simulink model "Kalman_offline"  (R2022b)
settings: Solver=VariableStepAuto  StartTime=0.0  StopTime=10.0  RelTol=1e-3
values from neighbouring files (symbols this model uses):
  A_d = (eye(size(A))+Ts*A)    [Kalman_offline.m]    (also in Main_sim.m; Startup_Script.m; Startup_labview.m; Test_ss.m)
  B_d = Ts*B    [Kalman_offline.m]    (also in Main_sim.m; Startup_Script.m; Startup_labview.m; Test_ss.m)
  bike_params = LoadBikeParameters(bike)    [Kalman_offline.m]    (also in Main_sim.m; Startup_Script.m; Startup_Script_v2.m; Startup_labview.m)
  C1 = [1 0 0 0 0 0 0 ... (first row only)    [Kalman_offline.m]    (also in Main_sim.m; Startup_Script.m; Startup_labview.m)
  C2 = [g+((-h_imu*g)/h) 0 (-h_imu*(h*v^2-(g*lr*c)))*sin(lambda)/((lr+lf)*h^2) + (v^2)*sin(lambda)/(lr+lf) 0 ... (first row only)    [Kalman_offline.m]    (also in Main_sim.m = [(-g+((-h_imu*g)/h)) 0 (-h_imu*(h*v^2-(g*lr*c)))*sin(lambda); Startup_Script.m = [(-g+((-h_imu*g)/h)) 0 (-h_imu*(h*v^2-(g*lr*c)))*sin(lambda); Startup_labview.m = [(g+((-h_imu*g)/h)) 0 (-h_imu*(h*v^2-(g*lr*c)))*sin(lambda)/)
  counter = (Ts_GPS / Ts) - 1    (= 9)    [Kalman_offline.m]    (also in Main_sim.m; Startup_Script.m; Startup_labview.m)
  D1 = [0 0 (-h_imu*lr*v)*sin(lambda)/((lr+lf)*h) 0 0 0 0]'    [Kalman_offline.m]    (also in Main_sim.m = [0 0 (-h_imu*lr*v)/((lr+lf)*h) 0 0 0 0]'; Startup_Script.m = [0 0 (-h_imu*lr*v)/((lr+lf)*h) 0 0 0 0]'; Startup_labview.m = [0 0 (-h_imu*lr*v)/((lr+lf)*h) 0 0 0 0]')
  D2 = [(-h_imu*lr*v)*sin(lambda)/((lr+lf)*h) 0 0 0 0]'    [Kalman_offline.m]    (also in Main_sim.m = [(-h_imu*lr*v)/((lr+lf)*h) 0 0 0 0]'; Startup_Script.m = [(-h_imu*lr*v)/((lr+lf)*h) 0 0 0 0]'; Startup_labview.m = [(-h_imu*lr*v)/((lr+lf)*h) 0 0 0 0]')
  initial_state_estimate = initial_state    [Main_sim.m]    (also in Startup_Script.m; Startup_Script_v2.m)
  Kalman_gain1 = Kalman_gain1'    [Kalman_offline.m]    (also in Main_sim.m; Startup_Script.m; Startup_labview.m)
  Kalman_gain2 = Kalman_gain2'    [Kalman_offline.m]    (also in Main_sim.m = Kalman_gain1(4:7,3:7); Startup_Script.m; Startup_labview.m = Kalman_gain1(4:7,3:7))
  lambda = bike_params.lambda_mod    [Kalman_offline.m]    (also in Main_sim.m; Startup_Script.m; Startup_Script_v2.m = bike_params.lambda; Startup_labview.m = bike_params.lambda)
  T = Rz*Ry*Rx    [Main_sim.m]    (also in Startup_Script.m)
  Ts = 0.01    [Kalman_offline.m]    (also in Main_sim.m; Startup_Script.m; Startup_Script_v2.m; Startup_labview.m)
  v = 3    [Main_sim.m]    (also in Startup_Script.m; Startup_Script_v2.m; Startup_labview.m = 2; Test_ss.m)
undefined symbols (not defined in the file or in its folder): initial_state
libraries: simulink x1
settings Model: Creator=gaizk  LastModifiedBy=gaizk

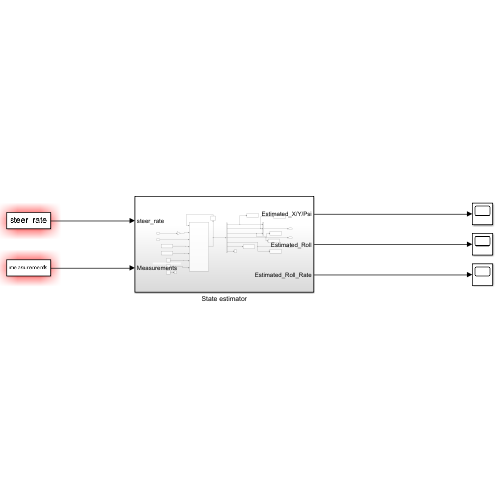
[thumbnail: Simulink's stored preview of the top-level diagram]
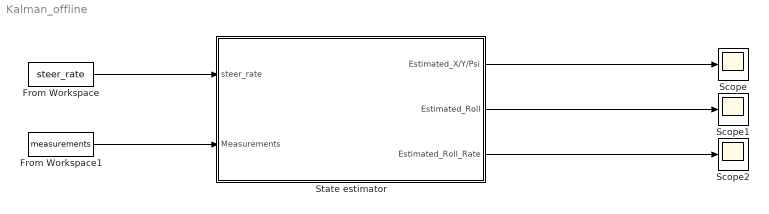
== system Kalman_offline ==
  From Workspace : FromWorkspace  VariableName=steer_rate
  From Workspace1 : FromWorkspace  VariableName=measurements
  Scope : Scope
  Scope1 : Scope
  Scope2 : Scope
  State estimator : Subsystem
  wires:
  From Workspace/1 -> State estimator/1(steer_rate)
  State estimator/1(Estimated_X/Y/Psi) -> Scope/1
  State estimator/2(Estimated_Roll) -> Scope1/1
  State estimator/3(Estimated_Roll_Rate) -> Scope2/1
  From Workspace1/1 -> State estimator/2(Measurements)

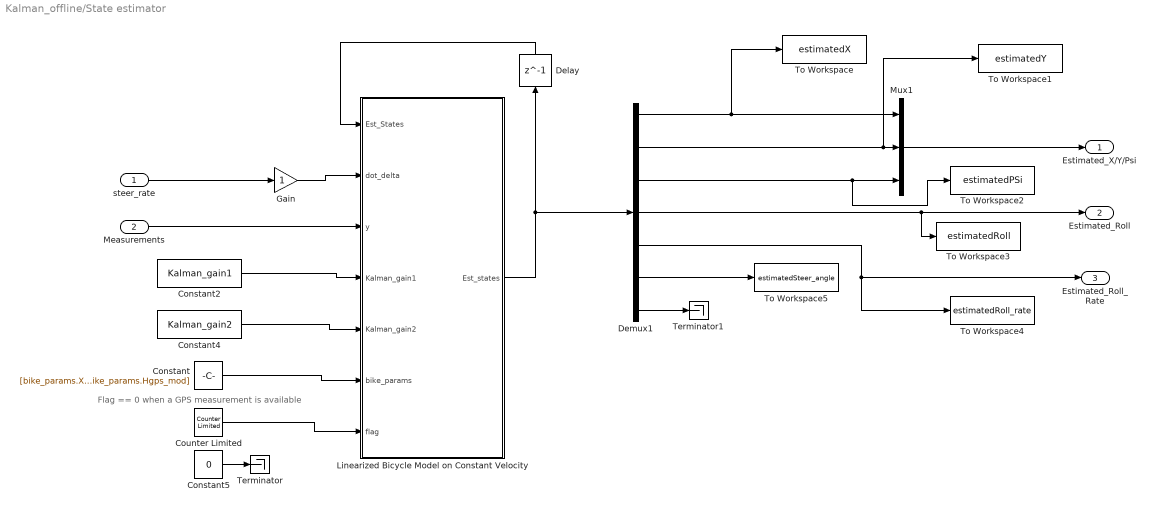
== system Kalman_offline/State estimator ==
  note: Flag == 0 when a GPS measurement is available
  steer_rate : Inport
  Measurements : Inport  Port=2
  Constant : Constant  Value=[bike_params.Xgps_mod bike_params.Ygps_mod bike_params.Hgps_mod]
  Constant2 : Constant  Value=Kalman_gain1  SampleTime=Ts
  Constant4 : Constant  Value=Kalman_gain2  SampleTime=Ts
  Constant5 : Constant  Value=0
  Counter Limited : simulink/Sources/Counter Limited  uplimit=counter  tsamp=Ts
  Delay : Delay  DelayLength=1  InitialCondition=[initial_state_estimate.x initial_state_estimate.y initial_state_estimate.heading initial_state.roll initial_state.roll_rate initial_state.steering v]  SampleTime=Ts
  Demux1 : Demux  Outputs=7
  Gain : Gain
  Linearized Bicycle Model on Constant Velocity : MATLAB Function  TreatAsAtomicUnit=on
  Mux1 : Mux  Inputs=3
  Terminator : Terminator
  Terminator1 : Terminator
  To Workspace : ToWorkspace  VariableName=estimatedX  SaveFormat=Timeseries  SampleTime=-1
  To Workspace1 : ToWorkspace  VariableName=estimatedY  SaveFormat=Timeseries  SampleTime=-1
  To Workspace2 : ToWorkspace  VariableName=estimatedPSi  SaveFormat=Timeseries  SampleTime=-1
  To Workspace3 : ToWorkspace  VariableName=estimatedRoll  SaveFormat=Timeseries  SampleTime=-1
  To Workspace4 : ToWorkspace  VariableName=estimatedRoll_rate  SaveFormat=Timeseries  SampleTime=-1
  To Workspace5 : ToWorkspace  VariableName=estimatedSteer_angle  SaveFormat=Timeseries  SampleTime=-1
  Estimated_X/Y/Psi : Outport  VectorParamsAs1DForOutWhenUnconnected=off
  Estimated_Roll : Outport  Port=2  VectorParamsAs1DForOutWhenUnconnected=off
  Estimated_Roll_Rate : Outport  Port=3  VectorParamsAs1DForOutWhenUnconnected=off
  wires:
  Linearized Bicycle Model on Constant Velocity/1(Est_states) -> Delay/1, Demux1/1
  Gain/1 -> Linearized Bicycle Model on Constant Velocity/2(dot_delta)
  Demux1/6 -> To Workspace5/1
  Demux1/5 -> Estimated_Roll_Rate/1, To Workspace4/1
  Delay/1 -> Linearized Bicycle Model on Constant Velocity/1(Est_States)
  steer_rate/1 -> Gain/1
  Demux1/2 -> To Workspace1/1, Mux1/2
  Demux1/1 -> To Workspace/1, Mux1/1
  Demux1/7 -> Terminator1/1
  Mux1/1 -> Estimated_X/Y/Psi/1
  Demux1/4 -> Estimated_Roll/1, To Workspace3/1
  Constant2/1 -> Linearized Bicycle Model on Constant Velocity/4(Kalman_gain1)
  Constant4/1 -> Linearized Bicycle Model on Constant Velocity/5(Kalman_gain2)
  Counter Limited/1 -> Linearized Bicycle Model on Constant Velocity/7(flag)
  Demux1/3 -> To Workspace2/1, Mux1/3
  Constant5/1 -> Terminator/1
  Constant/1 -> Linearized Bicycle Model on Constant Velocity/6(bike_params)
  Measurements/1 -> Linearized Bicycle Model on Constant Velocity/3(y)

== matlab function Kalman_offline/State estimator/Linearized Bicycle Model on Constant Velocity ==
  data: Est_States input; dot_delta input; y input; Kalman_gain1 input; Kalman_gain2 input; bike_params input; Est_states output; flag input; A_d parameter; B_d parameter; C1 parameter; C2 parameter; D1 parameter; D2 parameter; lambda parameter; T parameter
function Est_states  = fcn(Est_States, dot_delta, y, Kalman_gain1, Kalman_gain2, bike_params, flag, A_d, B_d, C1, C2, D1, D2, lambda, T)
% description 
% Inputs
%   Est_States := [X Y psi phi phi_dot delta v] are global at time t 
%   dot_delta_e := effective steering rate
%   y := measurement vector
%   Kalman_gain1 := Computed state_feedback gain including GPS meas
%   Kalman_gain2 := Computed state_feedback gain excluding GPS meas
%   bike_params := vector of bike parameters + gravity
%   Ts := Estimator sampling rate
%   v := constant velocity
%   flag := [0-1] increasing counter reseted at 1. When flag == 0 means
%           that GPS measurement is available
%
% Outputs
%   Est_states : = [X Y psi phi phi_dot delta v] global at time t+1


% Transform the states to local frame 
    Est_States_l = zeros(7,1);
    
    Est_States_l(1) = Est_States(1) * cos(Est_States(3)) + Est_States(2) * sin(Est_States(3));
    Est_States_l(2) = -Est_States(1) * sin(Est_States(3)) + Est_States(2) * cos(Est_States(3));
    Est_States_l(3) = 0;        % direction of bike is aligned with X local frame
    Est_States_l(4) = Est_States(4);
    Est_States_l(5) = Est_States(5);
    Est_States_l(6) = Est_States(6);
    Est_States_l(7) = Est_States(7);

% Transform measurements to local frame
    y_l = zeros(size(y));

    y_l(1) = y(1) * cos(Est_States(3)) + y(2) * sin(Est_States(3));
    y_l(2) = -y(1) * sin(Est_States(3)) + y(2) * cos(Est_States(3)); 
    y_l(3) = y(3);
    y_l(4) = y(4);
    y_l(5) = y(5);
    y_l(6) = y(6)*sin(lambda);
    y_l(7) = y(7);

% Correct for parameter values/sensor positions
% The parameters/positions are measures by us (can differ from true values)
X_gps_mod = bike_params(1);
Y_gps_mod = bike_params(2);
H_gps_mod = bike_params(3);

y_l(1) = y_l(1) - X_gps_mod;
y_l(2) = y_l(2) - Y_gps_mod - H_gps_mod*sin(Est_States(4));

% IMU correction
raw_acc  = [0 y_l(3) 0];
raw_gyro = [y_l(4) 0 y_l(5)];

% Apply the correction to the accelerometer measurement
acc_corr = T*raw_acc';

% Apply the correction to the gyro measurement
gyro_corr = T*raw_gyro';
% Results
y_l(3) =acc_corr(2) ;
y_l(4) =gyro_corr(1) ;
y_l(5) =gyro_corr(3) ;

% % Continuous Time update in local frame TODO: x(t+1) = (I+A delta_T)h_hat(t)
%     states_dot = zeros(7,1);
%     
%     states_dot(1) = Est_States(7);
%     states_dot(2) = v * (Est_States_l(3) + (lr/(lr+lf))*Est_States(6) );
%     states_dot(3) = (v/(lr+lf)) * Est_States(6);
%     states_dot(4) = Est_States(5);
%     states_dot(5) = (g/h)*Est_States(4) + ((v^2*h-lr*g*c)/(h^2*(lr+lf)))*Est_States(6) + ((lr*v)/(h*(lr+lf)))*dot_delta_e;
%     states_dot(6) = dot_delta_e;
%     states_dot(7) = 0;
% 
% % Discrete time update in local 
%     Est_States_l = Est_States_l + states_dot * Ts; 

% % C identity is used to see if the code runs
%     sen = zeros(6,1);
%     sen(1)      = States_l(1);  
%     sen(2)      = States_l(2);
%     %sen(3)      = States_l(3);
%     sen(3)      = States_l(4);
%     sen(4)      = States_l(5);
%     sen(5)      = States_l(6);
%     sen(6)      = States_l(7);

% % Transform measurements into local frame to see if code runs
%     meas_l = zeros(6,1);
%     meas_l(1) = meas(1) * cos(States(3)) + meas(2) * sin(States(3));
%     meas_l(2) = -meas(1) * sin(States(3)) + meas(2) * cos(States(3));
%     meas_l(3) = 0;
%     meas_l(3) = meas(3)-States(3);  
%     meas_l(3) = meas(4);
%     meas_l(4) = meas(5);
%     meas_l(5) = meas(6);
%     meas_l(6) = meas(7);
%     meas_l(7) = meas(7);

% Time update in local frame (from t to t+1)

    % Time update
     Est_States_l = A_d*Est_States_l + B_d*dot_delta;

    % Measurement update in local frame
     Est_states_l = zeros(7,1);

    % Sampling differentiation (Sensors rate 100Hz but GPS 10Hz)

    if flag == 0 % GPS sensors included
    
        % Select Kalman Gain
            K = Kalman_gain1;

        % Measurement prediction
            y_pred = C1*Est_States_l + D1*dot_delta;
    
        % Measurement update
            Est_states_l = Est_States_l + K * (y_l - y_pred);
        
    else % GPS sensors excluded
    
        % Select Kalman Gain
            K = Kalman_gain2;
    
        % Measurement prediction
            y_pred = C2*Est_States_l(4:7) + D2*dot_delta;
 
        % Measurement update
        Est_states_l(1) = Est_States_l(1);
        Est_states_l(2) = Est_States_l(2);
        Est_states_l(3) = Est_States_l(3);
        Est_states_l(4:7) = Est_States_l(4:7) + K * (y_l(3:7) - y_pred);

    end

    % states_l = Kalman_gain * (meas_l - sen);
    % states_l(1) = States_l(1) + Kalman_gain(1,1) * (meas_l(1) - x_m) + Kalman_gain(1,2) * (meas_l(2) - y_m) + Kalman_gain(1,3) * (meas_l(3) - psi_m) + Kalman_gain(1,4) * (meas_l(4) - phi_m) + Kalman_gain(1,5) * (meas_l(5) - dot_phi_m) + Kalman_gain(1,6) * (meas_l(6) - delta_m) + Kalman_gain(1,7) * (meas_l(7) - v_m);
    % states_l(2) = States_l(2) + Kalman_gain(2,1) * (meas_l(1) - x_m) + Kalman_gain(2,2) * (meas_l(2) - y_m) + Kalman_gain(2,3) * (meas_l(3) - psi_m) + Kalman_gain(2,4) * (meas_l(4) - phi_m) + Kalman_gain(2,5) * (meas_l(5) - dot_phi_m) + Kalman_gain(2,6) * (meas_l(6) - delta_m) + Kalman_gain(2,7) * (meas_l(7) - v_m);
    % states_l(3) = States_l(3) + Kalman_gain(3,1) * (meas_l(1) - x_m) + Kalman_gain(3,2) * (meas_l(2) - y_m) + Kalman_gain(3,3) * (meas_l(3) - psi_m) + Kalman_gain(3,4) * (meas_l(4) - phi_m) + Kalman_gain(3,5) * (meas_l(5) - dot_phi_m) + Kalman_gain(3,6) * (meas_l(6) - delta_m) + Kalman_gain(3,7) * (meas_l(7) - v_m);
    % states_l(4) = States_l(4) + Kalman_gain(4,1) * (meas_l(1) - x_m) + Kalman_gain(4,2) * (meas_l(2) - y_m) + Kalman_gain(4,3) * (meas_l(3) - psi_m) + Kalman_gain(4,4) * (meas_l(4) - phi_m) + Kalman_gain(4,5) * (meas_l(5) - dot_phi_m) + Kalman_gain(4,6) * (meas_l(6) - delta_m) + Kalman_gain(4,7) * (meas_l(7) - v_m);
    % states_l(5) = States_l(5) + Kalman_gain(5,1) * (meas_l(1) - x_m) + Kalman_gain(5,2) * (meas_l(2) - y_m) + Kalman_gain(5,3) * (meas_l(3) - psi_m) + Kalman_gain(5,4) * (meas_l(4) - phi_m) + Kalman_gain(5,5) * (meas_l(5) - dot_phi_m) + Kalman_gain(5,6) * (meas_l(6) - delta_m) + Kalman_gain(5,7) * (meas_l(7) - v_m);
    % states_l(6) = States_l(6) + Kalman_gain(6,1) * (meas_l(1) - x_m) + Kalman_gain(6,2) * (meas_l(2) - y_m) + Kalman_gain(6,3) * (meas_l(3) - psi_m) + Kalman_gain(6,4) * (meas_l(4) - phi_m) + Kalman_gain(6,5) * (meas_l(5) - dot_phi_m) + Kalman_gain(6,6) * (meas_l(6) - delta_m) + Kalman_gain(6,7) * (meas_l(7) - v_m);
    % states_l(7) = States_l(7) + Kalman_gain(7,1) * (meas_l(1) - x_m) + Kalman_gain(7,2) * (meas_l(2) - y_m) + Kalman_gain(7,3) * (meas_l(3) - psi_m) + Kalman_gain(7,4) * (meas_l(4) - phi_m) + Kalman_gain(7,5) * (meas_l(5) - dot_phi_m) + Kalman_gain(7,6) * (meas_l(6) - delta_m) + Kalman_gain(7,7) * (meas_l(7) - v_m);

% Transform to global the local states at time t+1 after measurement update
    Est_states = zeros(7,1);
    Est_states(3) = Est_States(3) + Est_states_l(3);    % direction update global
    
    % Change of Coordinates from local to global frame for  states 
    Est_states(1) = Est_states_l(1) * cos(Est_States(3)) - Est_states_l(2) * sin(Est_States(3));
    Est_states(2) = Est_states_l(1) * sin(Est_States(3)) + Est_states_l(2) * cos(Est_States(3));
    Est_states(4) = Est_states_l(4);
    Est_states(5) = Est_states_l(5);
    Est_states(6) = Est_states_l(6);
    Est_states(7) = Est_states_l(7);
    
    % Heading angle between pi and -pi
    Est_states(3) = wrapToPi(Est_states(3));

end
